simulink model "own_scout"  (R2018a)
settings: Solver=VariableStepAuto  StartTime=0.0  StopTime=500  FixedStep=0.01  RelTol=1e-5
libraries: simulink x2
settings Model: EnablePacing=on  Creator=daniel  LastModifiedBy=blond
settings SolverCC: ZeroCrossAlgorithm=Adaptive  AlgebraicLoopSolver=LineSearch
settings DebuggingCC: MaxConsecutiveZCsMsg=warning

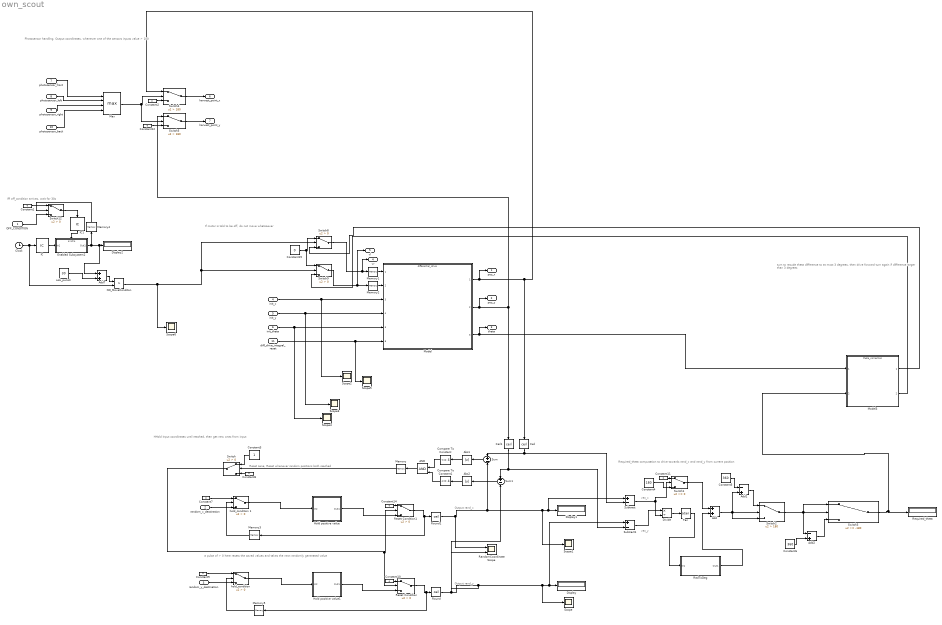
== system own_scout ==
  note: Photosensor handling. Output coordinates, whenever one of the sensors
      | inputs value > 100
  note: If motor is told to be off, do not move whatsoever
  note: turn to recude theta difference to at
      | most 3 degrees, then drive forward
      | turn again if difference larger than
      | 3 degrees
  note: Required_theta computation to drive towards rand_x and rand_y from current position
  note: vec_y
  note: Reset Lane, Reset whenever random positions both reached
  note: a pulse of > 0 here resets the saved values and takes the next randomly generated value
  note: Output rand_x
  note: HHold Input coordinates until reached, then get new ones from input
  note: Output rand_y
  note: vec_x
  note: Iff off_condition arrives, wait for 30s
  "OFF_CONDITION " : Inport  OutDataTypeStr=boolean
  random_x_destination : Inport  Port=2
  random_y_destination : Inport  Port=3
  "init_x " : Inport  Port=4
  init_y : Inport  Port=5
  "init_theta " : Inport  Port=6
  "photosensor_front " : Inport  Port=7
  photosensor_left : Inport  Port=8
  photosensor_right : Inport  Port=9
  photosensor_back : Inport  Port=10
  diff_drive_integral_reset : Inport  Port=11
  AND : Logic  IconShape=distinctive  AllPortsSameDT=off  OutDataTypeStr=boolean
  Abs1 : Abs
  Abs2 : Abs
  Add : Sum
  Add1 : Sum  Inputs=-+
  Add2 : Sum  Inputs=-+
  Add7 : Sum
  Ceil : Rounding  Operator=ceil
  Ceil1 : Rounding  Operator=ceil
  Clock : Clock
  Compare To Constant : simulink/Logic and Bit Operations/Compare To Constant  relop=<=  const=4  OutDataTypeStr=boolean
  Compare To Constant1 : simulink/Logic and Bit Operations/Compare To Constant  relop=<=  const=4  OutDataTypeStr=boolean
  Constant{1..2,7..12,14..15} (10 alike) : Constant  Value=0
  Constant3 : Constant
  Constant4 : Constant  Value=180
  Constant5 : Constant  Value=360
  Constant6 : Constant  Value=360
  Display : Display
  Display1 : Display
  Display2 : Display
  Divide : Product  Inputs=*/
  Enabled Subsystem2 : Subsystem  TreatAsAtomicUnit=on
  Hold positive value : Subsystem
  Hold positive value1 : Subsystem
  IC : InitialCondition  Value=-30
  IC1 : InitialCondition
  Max : MinMax  Function=max  Inputs=4
  Memory{,1..2,4} (4 alike) : Memory
  Memory3 : Memory  InheritSampleTime=on
  Memory5 : Memory  InheritSampleTime=on
  Model : ModelReference  ModelNameDialog=differential_drive.slx  SimulationMode=Normal  ModelReferenceVersion=1.313
  Model3 : ModelReference  ModelNameDialog=theta_correction.slx  SimulationMode=Normal  ModelReferenceVersion=1.8
  NO_MoveConditon : RelationalOperator  Operator=>  OutDataTypeStr=boolean  RndMeth=Simplest
  RadToDeg : Subsystem
  "RandomCoordinate Scope " : Scope  NumInputPorts=2
  Required_theta : Display
  Reset Condition : Switch  Criteria=u2 > Threshold
  Reset Condition1 : Switch  Criteria=u2 > Threshold
  Round : Rounding  Operator=ceil
  Round1 : Rounding  Operator=ceil
  Scope{,1..6} (7 alike) : Scope
  Subtract : Sum  Inputs=+-
  Subtract1 : Sum  Inputs=+-
  Sum : Sum  Inputs=+-
  Sum1 : Sum  Inputs=+-
  Switch{,8..9,12} (4 alike) : Switch  Criteria=u2 > Threshold
  Switch1 : Switch  ZeroCross=off
  Switch2 : Switch  Criteria=u2 > Threshold  Threshold=180  ZeroCross=off
  Switch3 : Switch  Threshold=-180  ZeroCross=off
  Switch4 : Switch  Criteria=u2 > Threshold  Threshold=180  ZeroCross=off
  Switch5 : Switch  Criteria=u2 > Threshold  Threshold=180  ZeroCross=off
  Tan : Trigonometry  Operator=atan  OutputSignalType=real
  "hold_condition " : Switch  Criteria=u2 > Threshold
  hold_condition 1 : Switch  Criteria=u2 > Threshold
  oob_punish : Constant  Value=30
  pos_x : Outport
  pos_y : Outport  Port=2
  theta : Outport  Port=3
  vr : Outport  Port=4
  vl : Outport  Port=5
  harvest_point_x : Outport  Port=6
  harvest_point_y : Outport  Port=7
  wires:
  "init_theta "/1 -> Scope4/1, Model/5
  init_y/1 -> Scope3/1, Model/4
  "init_x "/1 -> Scope2/1, Model/3
  Model/1 -> pos_x/1, Switch4/1, Ceil/1
  Model/2 -> pos_y/1, Ceil1/1, Switch5/1
  Model/3 -> Model3/1, theta/1
  diff_drive_integral_reset/1 -> Scope5/1, Model/6
  random_y_destination/1 -> "hold_condition "/3
  "hold_condition "/1 -> Hold positive value1/1(In2)
  Round/1 -> "RandomCoordinate Scope "/2, Sum1/2, Scope/1, Subtract1/1, Display/1
  Hold positive value1/1(Out1) -> Reset Condition/3
  Hold positive value/1(Out1) -> Reset Condition1/3
  hold_condition 1/1 -> Hold positive value/1(In2)
  random_x_destination/1 -> hold_condition 1/3
  Compare To Constant/1 -> AND/1
  Compare To Constant1/1 -> AND/2
  Ceil1/1 -> Sum1/1, Subtract1/2
  Ceil/1 -> Sum/1, Subtract/2
  AND/1 -> Memory/1
  Constant3/1 -> Switch/1
  Memory/1 -> Switch/2
  Switch/1 -> Reset Condition/2, Reset Condition1/2
  Subtract1/1 -> Divide/1
  Subtract/1 -> Switch1/2, Divide/2
  Divide/1 -> Tan/1
  Tan/1 -> RadToDeg/1(In1)
  Switch1/1 -> Add/1
  Constant4/1 -> Switch1/3
  Add/1 -> Switch2/3, Switch2/2, Add1/2
  Constant5/1 -> Add1/1
  Add1/1 -> Switch2/1
  Switch2/1 -> Switch3/1, Switch3/2, Add2/1
  Constant6/1 -> Add2/2
  Add2/1 -> Switch3/3
  Switch3/1 -> Model3/2, Required_theta/1
  RadToDeg/1(Out1) -> Add/2
  Constant8/1 -> Switch/3
  Constant10/1 -> Reset Condition/1
  Constant11/1 -> Switch1/1
  Constant14/1 -> Reset Condition1/1
  Reset Condition1/1 -> Memory3/1, Round1/1
  Reset Condition/1 -> Memory5/1, Round/1
  Sum/1 -> Abs1/1
  Abs1/1 -> Compare To Constant/1
  Abs2/1 -> Compare To Constant1/1
  Sum1/1 -> Abs2/1
  Memory5/1 -> "hold_condition "/2
  Memory3/1 -> hold_condition 1/2
  Constant9/1 -> "hold_condition "/1
  Constant15/1 -> Switch9/1, Switch8/1
  Switch8/1 -> vr/1, Memory1/1
  Switch9/1 -> Memory2/1, vl/1
  "photosensor_front "/1 -> Max/1
  photosensor_left/1 -> Max/2
  photosensor_right/1 -> Max/3
  photosensor_back/1 -> Max/4
  Max/1 -> Switch5/2, Switch4/2
  Switch4/1 -> harvest_point_x/1
  Switch5/1 -> harvest_point_y/1
  Constant7/1 -> hold_condition 1/1
  Round1/1 -> "RandomCoordinate Scope "/1, Scope1/1, Subtract/1, Display1/1, Sum/2
  Model3/2 -> Switch9/3
  Model3/1 -> Switch8/3
  Memory4/1 -> Switch12/2
  IC/1 -> Enabled Subsystem2/1(In1)
  IC1/1 -> Enabled Subsystem2/Enable
  Clock/1 -> NO_MoveConditon/2, IC/1
  Enabled Subsystem2/1(Out1) -> Memory4/1, Add7/1, Display2/1
  Switch12/1 -> IC1/1
  Add7/1 -> NO_MoveConditon/1
  "OFF_CONDITION "/1 -> Switch12/3
  oob_punish/1 -> Add7/2
  NO_MoveConditon/1 -> Switch8/2, Switch9/2, Scope6/1
  Memory1/1 -> Model/1
  Memory2/1 -> Model/2
  Constant1/1 -> Switch12/1
  Constant2/1 -> Switch4/3
  Constant12/1 -> Switch5/3

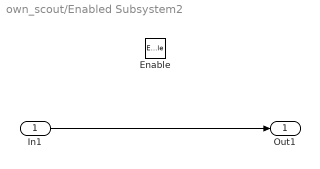
== system own_scout/Enabled Subsystem2 ==
  In1 : Inport
  Enable : EnablePort
  Out1 : Outport
  wires:
  In1/1 -> Out1/1

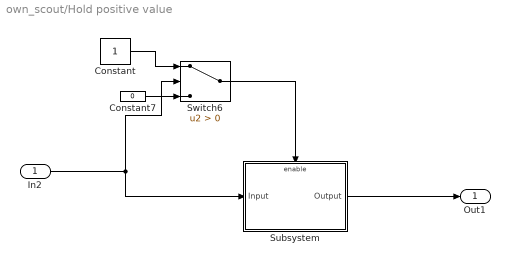
== system own_scout/Hold positive value ==
  In2 : Inport
  Constant : Constant
  Constant7 : Constant  Value=0
  Subsystem : Subsystem
  Switch6 : Switch  Criteria=u2 > Threshold
  Out1 : Outport
  wires:
  In2/1 -> Subsystem/1(Input), Switch6/2
  Switch6/1 -> Subsystem/Enable
  Constant/1 -> Switch6/1
  Subsystem/1(Output) -> Out1/1
  Constant7/1 -> Switch6/3

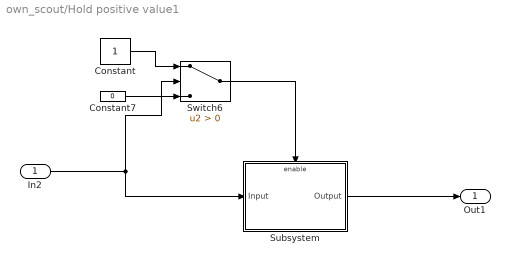
== system own_scout/Hold positive value1 ==
  In2 : Inport
  Constant : Constant
  Constant7 : Constant  Value=0
  Subsystem : Subsystem
  Switch6 : Switch  Criteria=u2 > Threshold
  Out1 : Outport
  wires:
  In2/1 -> Subsystem/1(Input), Switch6/2
  Switch6/1 -> Subsystem/Enable
  Constant/1 -> Switch6/1
  Subsystem/1(Output) -> Out1/1
  Constant7/1 -> Switch6/3

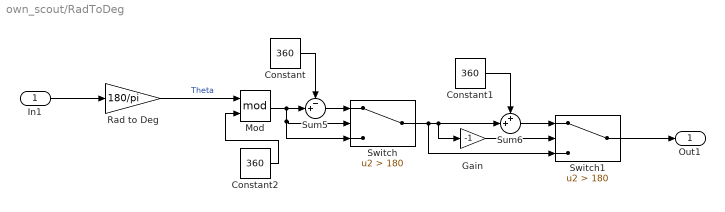
== system own_scout/RadToDeg ==
  In1 : Inport
  Constant : Constant  Value=360
  Constant1 : Constant  Value=360
  Constant2 : Constant  Value=360
  Gain : Gain  Gain=-1
  Mod : Math  Operator=mod  SaturateOnIntegerOverflow=on
  Rad to Deg : Gain  Gain=180/pi
  Sum5 : Sum  Inputs=-+|
  Sum6 : Sum  Inputs=++|
  Switch : Switch  Criteria=u2 > Threshold  Threshold=180
  Switch1 : Switch  Criteria=u2 > Threshold  Threshold=180
  Out1 : Outport
  wires:
  Constant/1 -> Sum5/1
  Constant1/1 -> Sum6/1
  Rad to Deg/1 -> Mod/1  "Theta"
  Gain/1 -> Switch1/2
  Switch/1 -> Sum6/2, Gain/1, Switch1/3
  Sum5/1 -> Switch/1
  Mod/1 -> Sum5/2, Switch/2, Switch/3
  Sum6/1 -> Switch1/1
  Constant2/1 -> Mod/2
  In1/1 -> Rad to Deg/1
  Switch1/1 -> Out1/1

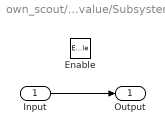
== system own_scout/Hold positive value/Subsystem ==
  Input : Inport
  Enable : EnablePort
  Output : Outport
  wires:
  Input/1 -> Output/1

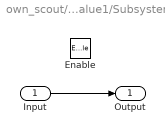
== system own_scout/Hold positive value1/Subsystem ==
  Input : Inport
  Enable : EnablePort
  Output : Outport
  wires:
  Input/1 -> Output/1
